simulink model "esercizio1"  (R2020a)
settings: Solver=VariableStepAuto  StartTime=0.0  StopTime=100  RelTol=1e-3
settings Model: Creator=bogda  LastModifiedBy=bogda

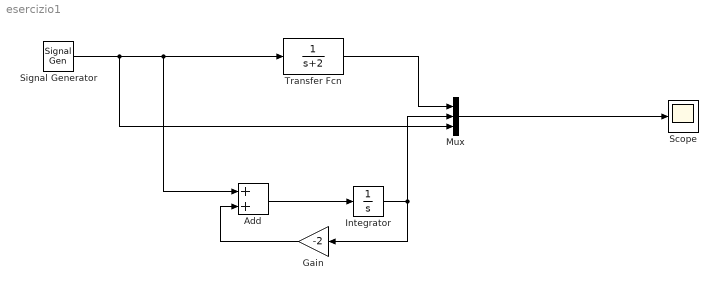
== system esercizio1 ==
  Add : Sum
  Gain : Gain  Gain=-2
  Integrator : Integrator  InitialCondition=2
  Mux : Mux  Inputs=3
  Scope : Scope
  Signal Generator : SignalGenerator  WaveForm=square  Units=rad/sec
  Transfer Fcn : TransferFcn  Denominator=[1 2]
  wires:
  Transfer Fcn/1 -> Mux/1
  Mux/1 -> Scope/1
  Add/1 -> Integrator/1
  Integrator/1 -> Mux/2, Gain/1
  Gain/1 -> Add/2
  Signal Generator/1 -> Mux/3, Add/1, Transfer Fcn/1
